simulink model "AEB_Project"  (R2021a)
settings: Solver=VariableStepAuto  StartTime=0.0  StopTime=17.0  RelTol=1e-3
values from neighbouring files (symbols this model uses):
  refPose = refPath.States    [PathPlanning_Step1.m]
libraries: robotalgslib x1, autolibshared x1, simulink x1
settings Model: Creator=USER  LastModifiedBy=USER

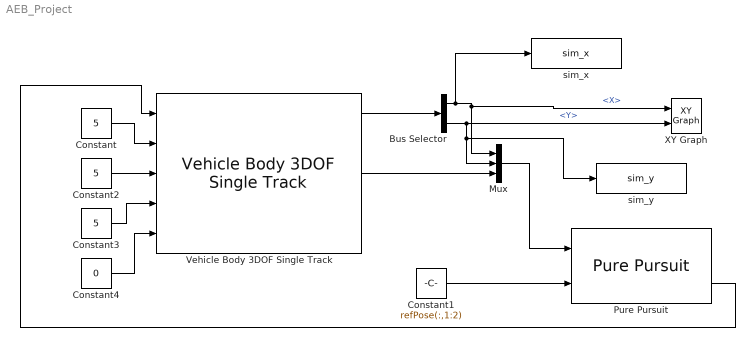
== system AEB_Project ==
  Bus Selector : BusSelector  OutputSignals=InertFrm.Cg.Disp.X,InertFrm.Cg.Disp.Y
  Constant : Constant  Value=5
  Constant1 : Constant  Value=refPose(:,1:2)
  Constant2 : Constant  Value=5
  Constant3 : Constant  Value=5
  Constant4 : Constant  Value=0
  Mux : Mux  Inputs=3
  Pure Pursuit : robotalgslib/Pure Pursuit  DesiredLinearVelocity=10  MaxAngularVelocity=1.0  LookaheadDistance=3  TargetDirPort=off  SimulateUsing=Code generation
  Vehicle Body 3DOF Single Track : autolibshared/Vehicle Body 3DOF Single Track  trackMode=Single (bicycle)  inputMode=External longitudinal velocity  frontSteerMode=on  rearSteerMode=off  windMode=off  muMode=off  extFMode=off  extMMode=off  htchFMode=off  htchMMode=off  extXo=on  extpsio=on  extxdoto=off  extro=off  extYo=on  extTamb=off  extydoto=off  aMode=2  NF=2  NR=2  m=2000  a=1.4  b=1.6  h=0.35  dh=1  hh=0.2  X_o=0  xdot_o=0  CalphaMode=off  sigmaMode=on  d=0  hl=0  w=[1.4,1.4]  Cy_f=12e3  Cy_r=11e3  sigma_f=.1  sigma_r=.1  alpha_f_brk=[-.1 .1]  Cy_f_data=[-9e3 9e3]  alpha_r_brk=[-.1 .1]  Cy_r_data=[-9e3 9e3]  Y_o=0  ydot_o=0  Izz=4000  psi_o=0  r_o=0  Af=2  Cd=.3  Cl=.1  Cpm=.1  beta_w=[0:0.01:0.3]  Cs=[0:0.03:0.9]  Cym=[0:0.01:0.3]  Pabs=101325  Tair=273  g=9.81  mu=1  xdot_tol=.01  Fznom=5000  Fxtire_sat=7e4  Fytire_sat=7e4  longOff=0  latOff=0  vertOff=0  wrapAng=off
      settings: SourceProductBaseCode=PW,DR,MT,UV,VE
  XY Graph : simulink/Sinks/XY Graph  xmin=0  xmax=60  ymin=0  ymax=60  st=-1
  sim_x : ToWorkspace  VariableName=sim_x  SampleTime=-1
  sim_y : ToWorkspace  VariableName=sim_y  SampleTime=-1
  wires:
  Constant/1 -> Vehicle Body 3DOF Single Track/2
  Vehicle Body 3DOF Single Track/1 -> Bus Selector/1
  Bus Selector/1 -> sim_x/1, XY Graph/1, Mux/1  "<X>"
  Bus Selector/2 -> sim_y/1, Mux/2, XY Graph/2  "<Y>"
  Vehicle Body 3DOF Single Track/4 -> Mux/3
  Mux/1 -> Pure Pursuit/1
  Constant1/1 -> Pure Pursuit/2
  Constant2/1 -> Vehicle Body 3DOF Single Track/3
  Constant3/1 -> Vehicle Body 3DOF Single Track/4
  Constant4/1 -> Vehicle Body 3DOF Single Track/5
  Pure Pursuit/2 -> Vehicle Body 3DOF Single Track/1
